simulink model "BLOC_Environment"  (R2016a)
settings: Solver=VariableStepAuto  StartTime=0.0  StopTime=10.0  RelTol=1e-3
undefined symbols (not defined in the file): hev_dt
settings Model: Creator=Florent  LastModifiedBy=Florent
settings OptimizationCC: DefaultParameterBehavior=Inlined  OptimizeModelRefInitCode=on  LifeSpan=1
settings RTWCC: SystemTargetFile=ert.tlc  TemplateMakefile=ert_default_tmf  GenerateReport=on  IncludeHyperlinkInReport=on  LaunchReport=on  TargetLang=C++  GenerateTraceInfo=on  GenerateTraceReport=on  GenerateTraceReportSl=on  GenerateTraceReportSf=on  GenerateTraceReportEml=on
settings CodeAppCC: ForceParamTrailComments=on  OperatorAnnotations=on  SimulinkDataObjDesc=on  SFDataObjDesc=on  MATLABFcnDesc=on  InsertBlockDesc=on  MATLABSourceComments=on
settings ERTTargetCC: GenerateSampleERTMain=on  MultiInstanceERTCode=on  CodeInterfacePackaging=C++ class  InlinedParameterPlacement=NonHierarchical  RootIOFormat=Structure reference  ERTCustomFileTemplate=example_file_process.tlc

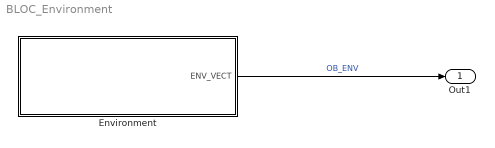
== system BLOC_Environment ==
  Environment : Subsystem  TreatAsAtomicUnit=on  SystemSampleTime=hev_dt
  Out1 : Outport  PortDimensions=3
  wires:
  Environment/1(ENV_VECT) -> Out1/1  "OB_ENV"

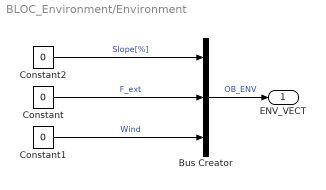
== system BLOC_Environment/Environment ==
  Bus Creator : BusCreator  Inputs=3
  Constant : Constant  Value=0
  Constant1 : Constant  Value=0
  Constant2 : Constant  Value=0
  ENV_VECT : Outport
  wires:
  Constant2/1 -> Bus Creator/1  "Slope[%]"
  Constant/1 -> Bus Creator/2  "F_ext"
  Constant1/1 -> Bus Creator/3  "Wind"
  Bus Creator/1 -> ENV_VECT/1  "OB_ENV"
